simulink model "CAN_Receiver"  (R2021a)
settings: Solver=VariableStepAuto  StartTime=0.0  StopTime=10.0  RelTol=1e-3
libraries: arduinolib x8
settings Model: Creator=departement-techniqu  LastModifiedBy=departement-techniqu

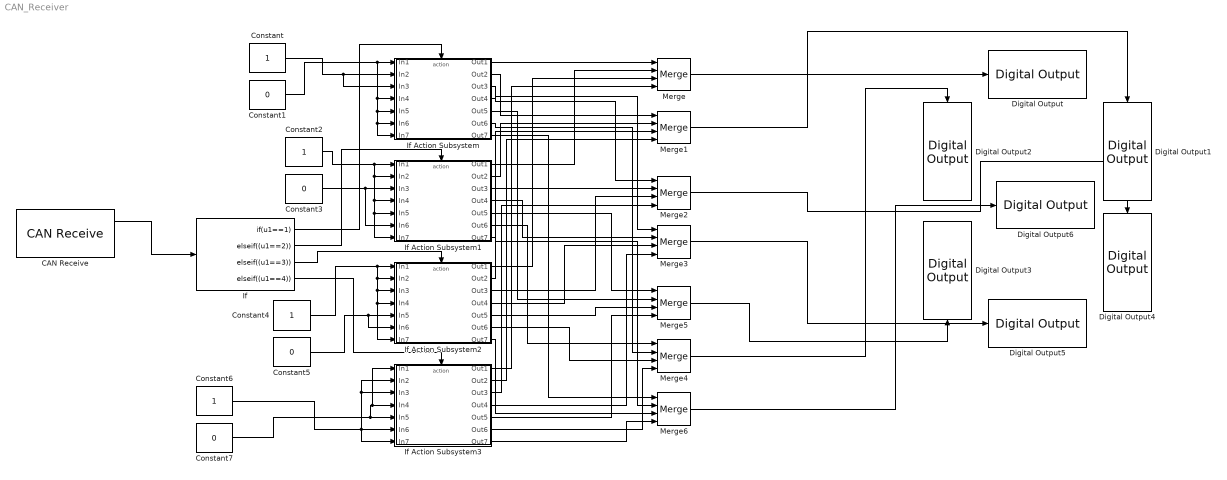
== system CAN_Receiver ==
  CAN Receive : arduinolib/CAN Receive  outputDataType=Raw data  identifierType=Standard (11-bit identifier)  messageId=100  msgLength=1  SampleTime=0.1  outputError=off  outputRemote=off
      settings: SourceProductBaseCode=ARDUINO
  Constant{,2,4,6} (4 alike) : Constant
  Constant{1,3,5,7} (4 alike) : Constant  Value=0
  Digital Output : arduinolib/Digital Output  pinNumber=1  Direction=output  blockPlatform=arduino
  Digital Output1 : arduinolib/Digital Output  pinNumber=2  Direction=output  blockPlatform=arduino
  Digital Output2 : arduinolib/Digital Output  pinNumber=6  Direction=output  blockPlatform=arduino
  Digital Output3 : arduinolib/Digital Output  pinNumber=5  Direction=output  blockPlatform=arduino
  Digital Output4 : arduinolib/Digital Output  pinNumber=3  Direction=output  blockPlatform=arduino
  Digital Output5 : arduinolib/Digital Output  pinNumber=4  Direction=output  blockPlatform=arduino
  Digital Output6 : arduinolib/Digital Output  pinNumber=7  Direction=output  blockPlatform=arduino
  If : If  IfExpression=u1==1  ElseIfExpressions=(u1==2),(u1==3),(u1==4)  ShowElse=off
  If Action Subsystem : Subsystem  TreatAsAtomicUnit=on
  If Action Subsystem1 : Subsystem  TreatAsAtomicUnit=on
  If Action Subsystem2 : Subsystem  TreatAsAtomicUnit=on
  If Action Subsystem3 : Subsystem  TreatAsAtomicUnit=on
  Merge{,1..6} (7 alike) : Merge  Inputs=4
  wires:
  CAN Receive/1 -> If/1
  Merge/1 -> Digital Output/1
  Merge1/1 -> Digital Output1/1
  Merge2/1 -> Digital Output4/1
  Merge3/1 -> Digital Output5/1
  Merge5/1 -> Digital Output3/1
  Merge4/1 -> Digital Output2/1
  Merge6/1 -> Digital Output6/1
  If Action Subsystem/1(Out1) -> Merge/1
  If Action Subsystem1/1(Out1) -> Merge/2
  If Action Subsystem2/1(Out1) -> Merge/3
  If Action Subsystem3/1(Out1) -> Merge/4
  If Action Subsystem/2(Out2) -> Merge1/1
  If Action Subsystem1/2(Out2) -> Merge1/2
  If Action Subsystem2/2(Out2) -> Merge1/3
  If Action Subsystem3/2(Out2) -> Merge1/4
  If Action Subsystem/3(Out3) -> Merge2/1
  If Action Subsystem1/3(Out3) -> Merge2/2
  If Action Subsystem2/3(Out3) -> Merge2/3
  If Action Subsystem3/3(Out3) -> Merge2/4
  If Action Subsystem/4(Out4) -> Merge3/1
  If Action Subsystem1/4(Out4) -> Merge3/2
  If Action Subsystem2/4(Out4) -> Merge3/3
  If Action Subsystem3/4(Out4) -> Merge3/4
  If Action Subsystem1/5(Out5) -> Merge5/1
  If Action Subsystem/5(Out5) -> Merge5/2
  If Action Subsystem2/5(Out5) -> Merge5/3
  If Action Subsystem3/5(Out5) -> Merge5/4
  If Action Subsystem/6(Out6) -> Merge4/2
  If Action Subsystem1/6(Out6) -> Merge4/1
  If Action Subsystem2/6(Out6) -> Merge4/3
  If Action Subsystem3/6(Out6) -> Merge4/4
  If Action Subsystem/7(Out7) -> Merge6/1
  If Action Subsystem1/7(Out7) -> Merge6/2
  If Action Subsystem2/7(Out7) -> Merge6/3
  If Action Subsystem3/7(Out7) -> Merge6/4
  If/1 -> If Action Subsystem/Action
  If/2 -> If Action Subsystem1/Action
  If/3 -> If Action Subsystem2/Action
  If/4 -> If Action Subsystem3/Action
  Constant/1 -> If Action Subsystem/3(In3), If Action Subsystem/2(In2)
  Constant1/1 -> If Action Subsystem/7(In7), If Action Subsystem/6(In6), If Action Subsystem/5(In5), If Action Subsystem/4(In4), If Action Subsystem/1(In1)
  Constant2/1 -> If Action Subsystem1/4(In4), If Action Subsystem1/5(In5), If Action Subsystem1/7(In7), If Action Subsystem1/2(In2), If Action Subsystem1/1(In1)
  Constant3/1 -> If Action Subsystem1/6(In6), If Action Subsystem1/3(In3)
  Constant4/1 -> If Action Subsystem2/7(In7), If Action Subsystem2/4(In4), If Action Subsystem2/3(In3), If Action Subsystem2/2(In2), If Action Subsystem2/1(In1)
  Constant5/1 -> If Action Subsystem2/6(In6), If Action Subsystem2/5(In5)
  Constant6/1 -> If Action Subsystem3/3(In3), If Action Subsystem3/2(In2), If Action Subsystem3/7(In7), If Action Subsystem3/6(In6)
  Constant7/1 -> If Action Subsystem3/1(In1), If Action Subsystem3/4(In4), If Action Subsystem3/5(In5)

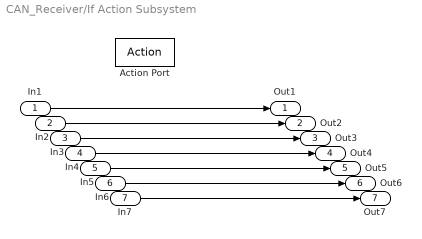
== system CAN_Receiver/If Action Subsystem ==
  In1 : Inport
  In2 : Inport  Port=2
  In3 : Inport  Port=3
  In4 : Inport  Port=4
  In5 : Inport  Port=5
  In6 : Inport  Port=6
  In7 : Inport  Port=7
  Action Port : ActionPort  ActionPortLabel=if(u1==1)
  Out1 : Outport
  Out2 : Outport  Port=2
  Out3 : Outport  Port=3
  Out4 : Outport  Port=4
  Out5 : Outport  Port=5
  Out6 : Outport  Port=6
  Out7 : Outport  Port=7
  wires:
  In1/1 -> Out1/1
  In2/1 -> Out2/1
  In3/1 -> Out3/1
  In4/1 -> Out4/1
  In5/1 -> Out5/1
  In6/1 -> Out6/1
  In7/1 -> Out7/1

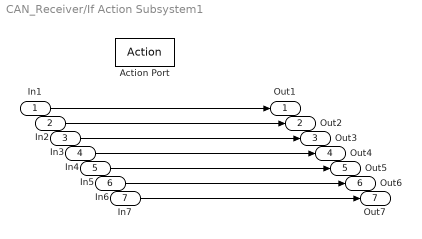
== system CAN_Receiver/If Action Subsystem1 ==
  In1 : Inport
  In2 : Inport  Port=2
  In3 : Inport  Port=3
  In4 : Inport  Port=4
  In5 : Inport  Port=5
  In6 : Inport  Port=6
  In7 : Inport  Port=7
  Action Port : ActionPort  ActionPortLabel=elseif((u1==2))
  Out1 : Outport
  Out2 : Outport  Port=2
  Out3 : Outport  Port=3
  Out4 : Outport  Port=4
  Out5 : Outport  Port=5
  Out6 : Outport  Port=6
  Out7 : Outport  Port=7
  wires:
  In1/1 -> Out1/1
  In2/1 -> Out2/1
  In3/1 -> Out3/1
  In4/1 -> Out4/1
  In5/1 -> Out5/1
  In6/1 -> Out6/1
  In7/1 -> Out7/1

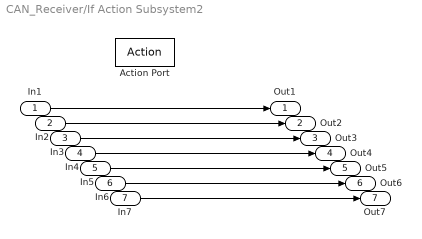
== system CAN_Receiver/If Action Subsystem2 ==
  In1 : Inport
  In2 : Inport  Port=2
  In3 : Inport  Port=3
  In4 : Inport  Port=4
  In5 : Inport  Port=5
  In6 : Inport  Port=6
  In7 : Inport  Port=7
  Action Port : ActionPort  ActionPortLabel=elseif((u1==3))
  Out1 : Outport
  Out2 : Outport  Port=2
  Out3 : Outport  Port=3
  Out4 : Outport  Port=4
  Out5 : Outport  Port=5
  Out6 : Outport  Port=6
  Out7 : Outport  Port=7
  wires:
  In1/1 -> Out1/1
  In2/1 -> Out2/1
  In3/1 -> Out3/1
  In4/1 -> Out4/1
  In5/1 -> Out5/1
  In6/1 -> Out6/1
  In7/1 -> Out7/1

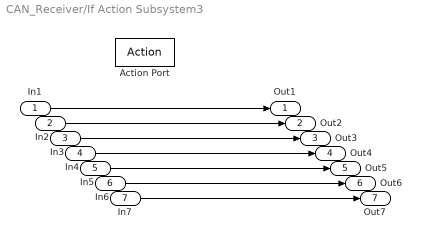
== system CAN_Receiver/If Action Subsystem3 ==
  In1 : Inport
  In2 : Inport  Port=2
  In3 : Inport  Port=3
  In4 : Inport  Port=4
  In5 : Inport  Port=5
  In6 : Inport  Port=6
  In7 : Inport  Port=7
  Action Port : ActionPort  ActionPortLabel=elseif((u1==4))
  Out1 : Outport
  Out2 : Outport  Port=2
  Out3 : Outport  Port=3
  Out4 : Outport  Port=4
  Out5 : Outport  Port=5
  Out6 : Outport  Port=6
  Out7 : Outport  Port=7
  wires:
  In1/1 -> Out1/1
  In2/1 -> Out2/1
  In3/1 -> Out3/1
  In4/1 -> Out4/1
  In5/1 -> Out5/1
  In6/1 -> Out6/1
  In7/1 -> Out7/1
